simulink model "closed_loop"  (R2016b)
settings: Solver=FixedStepAuto  StartTime=0.0  StopTime=10  FixedStep=1/100  RelTol=1e-3  AbsTol=1e-3
model workspace: external: MATLAB File params.m (data not in the file)
undefined symbols (not defined in the file or in its folder): b, g, k, m
libraries: nesl_utility x7
settings Model: Creator=Jocke  LastModifiedBy=frehage
settings OptimizationCC: UseDivisionForNetSlopeComputation=on
settings RTWCC: Toolchain=GNU gcc/g++ v4.4.x | gmake (64-bit Linux)
settings SimscapeCC: SimscapeLogType=all  SimscapeLogDataHistory=10000

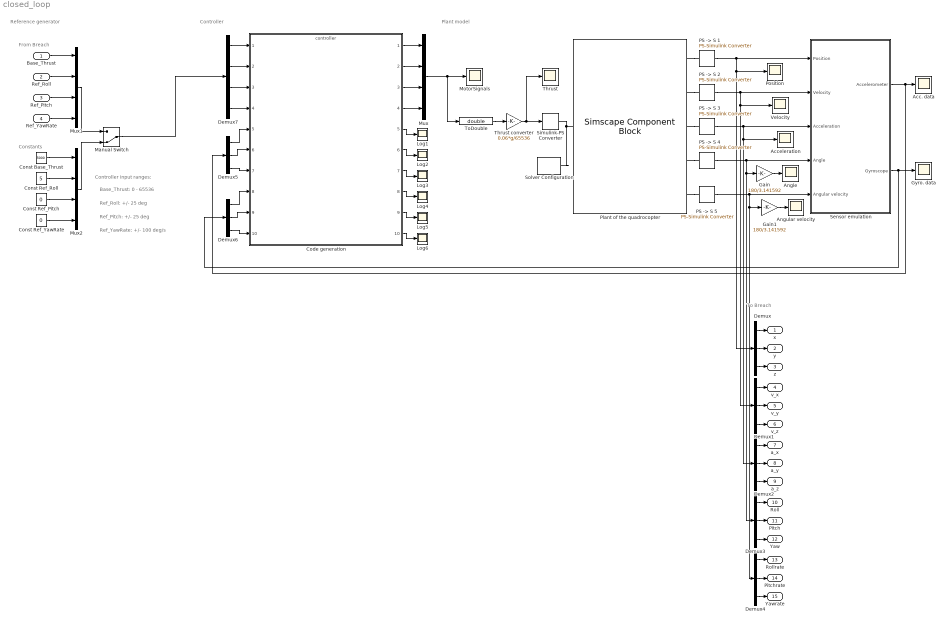
== system closed_loop ==
  note: To Breach
  note: From Breach
  note: Plant model
  note: Controller
  note: Constants
  note: Reference generator
  note: Ref_Roll: +/- 25 deg
  note: Base_Thrust: 0 - 65536
  note: Ref_Pitch: +/- 25 deg
  note: Ref_YawRate: +/- 100 deg/s
  note: Controller input ranges:
  Base_Thrust : Inport  OutDataTypeStr=double
  Ref_Roll : Inport  Port=2  OutDataTypeStr=double
  Ref_Pitch : Inport  Port=3  OutDataTypeStr=double
  Ref_YawRate : Inport  Port=4  OutDataTypeStr=double
  Acc. data : Scope
  Acceleration : Scope
  Angle : Scope
  Angular velocity : Scope
  Code generation : ModelReference  ModelNameDialog=controller.slx  SimulationMode=Normal  ModelReferenceVersion=1.162
  Const Base_Thrust : Constant  Value=5000
  Const Ref_Pitch : Constant  Value=0
  Const Ref_Roll : Constant  Value=5
  Const Ref_YawRate : Constant  Value=0
  Demux{,1..6} (7 alike) : Demux  Outputs=3
  Demux7 : Demux
  Gain : Gain  Gain=180/3.141592
  Gain1 : Gain  Gain=180/3.141592
  Gyro. data : Scope
  Log{1..6} (6 alike) : Scope
  Manual Switch : ManualSwitch  CurrentSetting=0
  MotorSignals : Scope
  Mux : Mux
  Mux1 : Mux
  Mux2 : Mux
  PS -> S {1..5} (5 alike) : nesl_utility/PS-Simulink Converter  PhysicalDomain=network_engine_domain  SubClassName=ps_output  LeftPortType=input  RightPortType=output  PseudoPeriodic=off  Frequencies=[]  Unit=1  AffineConversion=off
  Plant of the quadrocopter : SimscapeComponentBlock  SourceFile=plant  ComponentPath=plant  ComponentVariants=plant  ComponentVariantNames=plant  ClassName=plant  SchemaVersion=1  m=m kg  g=g m/s^2  d=d m  k=b  b=k
      settings: CopyFcn=simscape.engine.sli.internal.componentblockcallback(gcbh,'COPY')  PreCopyFcn=simscape.engine.sli.internal.componentblockcallback(gcbh,'PRECOPY')  PreDeleteFcn=simscape.engine.sli.internal.componentblockcallback(gcbh,'PREDELETE')
      mask Type: Plant of quadrocopter
      mask Display:
      | disp('Simscape\n\n\n')
      | disp('\n\n\nplant');
      | color('red');
      | port_label('RConn', 5,'Angular velocity');
      | port_label('RConn', 4,'Angle');
      | port_label('RConn', 3,'Acceleration');
      | port_label('RConn', 2,'Velocity');
      | port_label('RConn', 1,'Position');
      | port_label('LConn', 1,'Thrust');
  Position : Scope
  Sensor emulation : Subsystem
  Simulink-PS Converter : nesl_utility/Simulink-PS Converter  PhysicalDomain=network_engine_domain  SubClassName=ps_input  LeftPortType=input  RightPortType=output  PseudoPeriodic=off  Frequencies=[]  NoiseDistribution=none  NoiseParameters=[]  Unit=1  AffineConversion=off  InputFiltering=off  SimscapeFilterOrder=1  InputFilterTimeConstant=0.001  UdotUserProvided=1
  Solver Configuration : nesl_utility/Solver Configuration  PhysicalDomain=network_engine_domain  SubClassName=solver  LeftPortType=input  RightPortType=generic  Accelerate=off  Tones=[]  Harmonics=[]  SimulateNoise=off  Profile=off  UseLocalSampling=off  EnableSwitchedLinearOptims=on  FrequencyDomain=off  UseCCode=off  RelTol=0.001  AbsTol=1e-06  MinStep=1e-09  ToWorkspace=off  RevertToSquareIcSolve=off  NumHomotopyIterations=100  PhasorMode=off  PhasorModeNumHarmonics=1  OverrideAbsTol=off  DoDC=off  ResidualTolerance=1e-09  UseLocalSolver=off  LocalSolverChoice=NE_BACKWARD_EULER_ADVANCER  LocalSolverSampleTime=0.001  DoFixedCost=off  MaxNonlinIter=3  MaxModeIter=2  LinearAlgebra=Sparse  DelaysMemoryBudget=1024  AutomaticFiltering=on  FilteringTimeConstant=0.001
  Thrust : Scope
  Thrust converter : Gain  Gain=0.06*g/65536
  ToDouble : DataTypeConversion  OutDataTypeStr=double  RndMeth=Round  SaturateOnIntegerOverflow=on
  Velocity : Scope
  x : Outport
  y : Outport  Port=2
  z : Outport  Port=3
  v_x : Outport  Port=4
  v_y : Outport  Port=5
  v_z : Outport  Port=6
  a_x : Outport  Port=7
  a_y : Outport  Port=8
  a_z : Outport  Port=9
  Roll : Outport  Port=10
  Pitch : Outport  Port=11
  Yaw : Outport  Port=12
  Rollrate : Outport  Port=13
  Pitchrate : Outport  Port=14
  Yawrate : Outport  Port=15
  wires:
  Code generation/1 -> Mux/1
  Code generation/4 -> Mux/4
  Code generation/3 -> Mux/3
  Code generation/2 -> Mux/2
  "PS -> S 5"/1 -> Gain1/1, Demux4/1, Sensor emulation/5(Angular velocity)
  "PS -> S 4"/1 -> Gain/1, Demux3/1, Sensor emulation/4(Angle)
  "PS -> S 3"/1 -> Sensor emulation/3(Acceleration), Demux2/1, Acceleration/1
  "PS -> S 2"/1 -> Sensor emulation/2(Velocity), Demux1/1, Velocity/1
  Demux/1 -> x/1
  Demux/2 -> y/1
  Demux/3 -> z/1
  Demux1/1 -> v_x/1
  Demux1/2 -> v_y/1
  Demux1/3 -> v_z/1
  Demux3/1 -> Roll/1
  Demux3/2 -> Pitch/1
  Demux3/3 -> Yaw/1
  Demux4/1 -> Rollrate/1
  Demux4/2 -> Pitchrate/1
  Demux4/3 -> Yawrate/1
  Demux2/1 -> a_x/1
  Demux2/2 -> a_y/1
  Demux2/3 -> a_z/1
  Demux5/1 -> Code generation/5
  Demux5/2 -> Code generation/6
  Demux5/3 -> Code generation/7
  Demux6/1 -> Code generation/8
  Demux6/2 -> Code generation/9
  Demux6/3 -> Code generation/10
  Sensor emulation/2(Gyroscope) -> Demux6/1, Gyro. data/1
  Sensor emulation/1(Accelerometer) -> Acc. data/1, Demux5/1
  Code generation/5 -> Log1/1
  Code generation/6 -> Log2/1
  Code generation/7 -> Log3/1
  Code generation/8 -> Log4/1
  Code generation/9 -> Log5/1
  Code generation/10 -> Log6/1
  Mux/1 -> MotorSignals/1, ToDouble/1
  Base_Thrust/1 -> Mux1/1
  Ref_Roll/1 -> Mux1/2
  Ref_Pitch/1 -> Mux1/3
  Ref_YawRate/1 -> Mux1/4
  Mux1/1 -> Manual Switch/1
  Const Base_Thrust/1 -> Mux2/1
  Const Ref_Roll/1 -> Mux2/2
  Const Ref_Pitch/1 -> Mux2/3
  Const Ref_YawRate/1 -> Mux2/4
  Mux2/1 -> Manual Switch/2
  Manual Switch/1 -> Demux7/1
  Demux7/1 -> Code generation/1
  Demux7/2 -> Code generation/2
  Demux7/3 -> Code generation/3
  Demux7/4 -> Code generation/4
  "PS -> S 1"/1 -> Demux/1, Position/1, Sensor emulation/1(Position)
  Gain/1 -> Angle/1
  Gain1/1 -> Angular velocity/1
  ToDouble/1 -> Thrust converter/1
  Thrust converter/1 -> Thrust/1, Simulink-PS Converter/1
  connections:
  Simulink-PS Converter/RConn1 -- Solver Configuration/RConn1 -- Plant of the quadrocopter/LConn1
  Plant of the quadrocopter/RConn1 -- "PS -> S 1"/LConn1
  Plant of the quadrocopter/RConn2 -- "PS -> S 2"/LConn1
  Plant of the quadrocopter/RConn3 -- "PS -> S 3"/LConn1
  Plant of the quadrocopter/RConn4 -- "PS -> S 4"/LConn1
  Plant of the quadrocopter/RConn5 -- "PS -> S 5"/LConn1

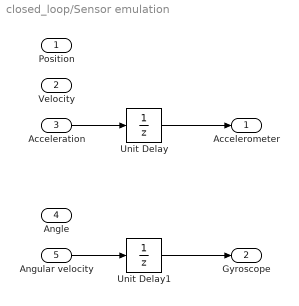
== system closed_loop/Sensor emulation ==
  Position : Inport  OutDataTypeStr=double  PortDimensions=3
  Velocity : Inport  Port=2  OutDataTypeStr=double  PortDimensions=3
  Acceleration : Inport  Port=3  OutDataTypeStr=double  PortDimensions=3
  Angle : Inport  Port=4  OutDataTypeStr=double  PortDimensions=3
  Angular velocity : Inport  Port=5  OutDataTypeStr=double  PortDimensions=3
  Unit Delay : UnitDelay  SampleTime=-1
  Unit Delay1 : UnitDelay  SampleTime=-1
  Accelerometer : Outport
  Gyroscope : Outport  Port=2
  wires:
  Acceleration/1 -> Unit Delay/1
  Unit Delay/1 -> Accelerometer/1
  Angular velocity/1 -> Unit Delay1/1
  Unit Delay1/1 -> Gyroscope/1
